simulink model "PI_Control"  (R2015a)
settings: Solver=ode45  StartTime=0.0  StopTime=10.0  RelTol=1e-3
undefined symbols (not defined in the file): kI, kp
libraries: simulink x1
settings Model: CovSFcnEnable=off  Creator=Rane  LastModifiedBy=brownsr
settings DebuggingCC: SolverPrmCheckMsg=warning

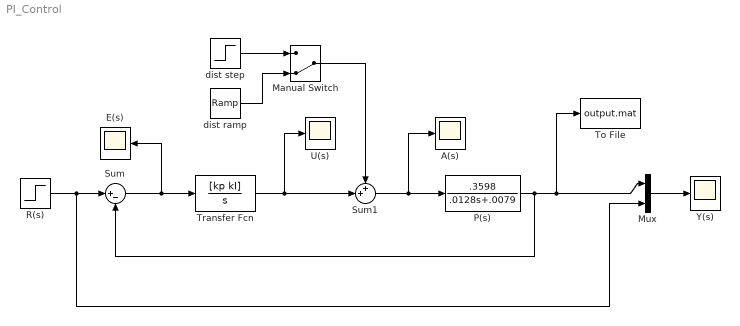
== system PI_Control ==
  A(s) : Scope
      settings: SaveName=ScopeData3
  E(s) : Scope
  Manual Switch : ManualSwitch  CurrentSetting=0
  Mux : Mux  Inputs=2
  P(s) : TransferFcn  Numerator=[.3598]  Denominator=[.0128 .0079]
  R(s) : Step  After=6.28  SampleTime=0
  Sum : Sum  Inputs=|+-
  Sum1 : Sum  Inputs=++|
  To File : ToFile  Filename=output.mat  MatrixName=vel
  Transfer Fcn : TransferFcn  Numerator=[kp kI]  Denominator=[1 0]
  U(s) : Scope
      settings: SaveName=ScopeData2
  Y(s) : Scope
      settings: ShowLegends=on
  dist ramp : simulink/Sources/Ramp  slope=1  start=0  X0=0
  dist step : Step  SampleTime=0
  wires:
  Sum1/1 -> A(s)/1, P(s)/1
  P(s)/1 -> To File/1, Mux/1, Sum/2
  Sum/1 -> Transfer Fcn/1, E(s)/1
  Transfer Fcn/1 -> U(s)/1, Sum1/2
  R(s)/1 -> Mux/2, Sum/1
  Mux/1 -> Y(s)/1
  Manual Switch/1 -> Sum1/1
  dist step/1 -> Manual Switch/1
  dist ramp/1 -> Manual Switch/2
